simulink model "curent_rotoric"  (R2022b)
settings: Solver=VariableStepAuto  StartTime=0.0  StopTime=10.0  RelTol=1e-3
values from neighbouring files (symbols this model uses):
  k = 0.035    [run_first.m]
settings Model: Creator=fabian  LastModifiedBy=fabian

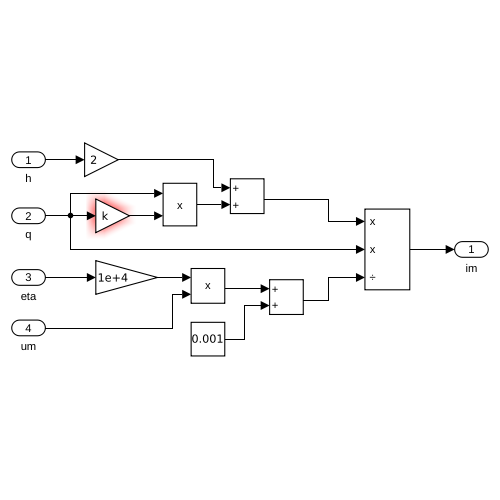
[thumbnail: Simulink's stored preview of the top-level diagram]
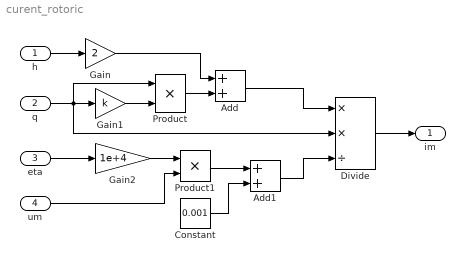
== system curent_rotoric ==
  h : Inport
  q : Inport  Port=2
  eta : Inport  Port=3
  um : Inport  Port=4
  Add : Sum
  Add1 : Sum
  Constant : Constant  Value=0.001
  Divide : Product  Inputs=**/
  Gain : Gain  Gain=2
  Gain1 : Gain  Gain=k
  Gain2 : Gain  Gain=1e+4
  Product : Product
  Product1 : Product
  im : Outport
  wires:
  h/1 -> Gain/1
  q/1 -> Gain1/1, Product/1, Divide/2
  eta/1 -> Gain2/1
  Gain2/1 -> Product1/1
  um/1 -> Product1/2
  Gain1/1 -> Product/2
  Constant/1 -> Add1/2
  Product/1 -> Add/2
  Gain/1 -> Add/1
  Add/1 -> Divide/1
  Add1/1 -> Divide/3
  Divide/1 -> im/1
  Product1/1 -> Add1/1
